simulink model "LAB3_SIMULINK_NO1_EBORA"  (R2023b)
settings: Solver=VariableStepAuto  StartTime=0.0  StopTime=20  RelTol=1e-3
values from neighbouring files (symbols this model uses):
  G1_den = [1 0 0]    [LAB3_MATLAB_NO1_BUENAFE.m]    (also in LAB3_MATLAB_NO2_RAGO.m)
  G1_num = [1]    [LAB3_MATLAB_NO1_BUENAFE.m]    (also in LAB3_MATLAB_NO2_RAGO.m)
  G2_den = [1 1]    [LAB3_MATLAB_NO1_BUENAFE.m]    (also in LAB3_MATLAB_NO2_RAGO.m)
  G2_num = [1]    [LAB3_MATLAB_NO1_BUENAFE.m]    (also in LAB3_MATLAB_NO2_RAGO.m)
  G3_den = [1 0]    [LAB3_MATLAB_NO1_BUENAFE.m]    (also in LAB3_MATLAB_NO2_RAGO.m)
  G3_num = [1]    [LAB3_MATLAB_NO1_BUENAFE.m]    (also in LAB3_MATLAB_NO2_RAGO.m)
  H1_den = [1 0]    [LAB3_MATLAB_NO1_BUENAFE.m]    (also in LAB3_MATLAB_NO2_RAGO.m)
  H1_num = [1]    [LAB3_MATLAB_NO1_BUENAFE.m]    (also in LAB3_MATLAB_NO2_RAGO.m)
  H2_den = [1 -1]    [LAB3_MATLAB_NO1_BUENAFE.m]    (also in LAB3_MATLAB_NO2_RAGO.m)
  H2_num = [1]    [LAB3_MATLAB_NO1_BUENAFE.m]    (also in LAB3_MATLAB_NO2_RAGO.m)
  H3_den = [1 -2]    [LAB3_MATLAB_NO1_BUENAFE.m]    (also in LAB3_MATLAB_NO2_RAGO.m)
  H3_num = [1]    [LAB3_MATLAB_NO1_BUENAFE.m]    (also in LAB3_MATLAB_NO2_RAGO.m)
  TF_den = conv(TF_num_down,TF_den_up)    [LAB3_MATLAB_NO1_BUENAFE.m]    (also in LAB3_MATLAB_NO2_RAGO.m)
  TF_num = conv(TF_num_up,TF_den_down)    [LAB3_MATLAB_NO1_BUENAFE.m]    (also in LAB3_MATLAB_NO2_RAGO.m)
settings Model: Creator=Troy  LastModifiedBy=Troy

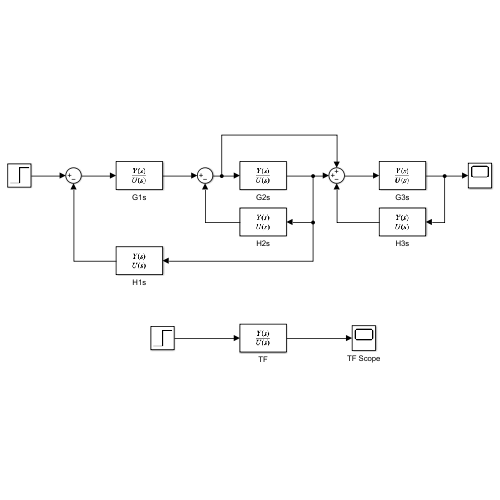
[thumbnail: Simulink's stored preview of the top-level diagram]
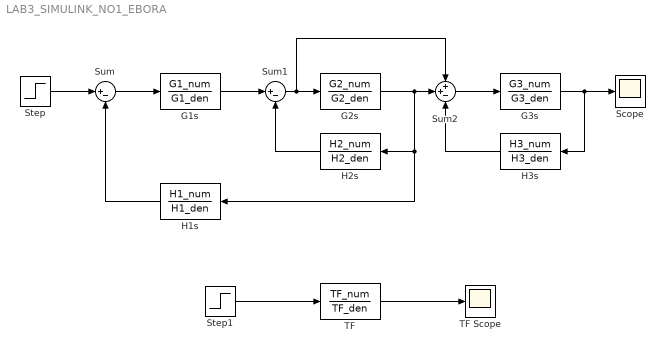
== system LAB3_SIMULINK_NO1_EBORA ==
  G1s : TransferFcn  Numerator=G1_num  Denominator=G1_den
  G2s : TransferFcn  Numerator=G2_num  Denominator=G2_den
  G3s : TransferFcn  Numerator=G3_num  Denominator=G3_den
  H1s : TransferFcn  Numerator=H1_num  Denominator=H1_den
  H2s : TransferFcn  Numerator=H2_num  Denominator=H2_den
  H3s : TransferFcn  Numerator=H3_num  Denominator=H3_den
  Scope : Scope
  Step : Step  Time=0  SampleTime=0
  Step1 : Step  Time=0  SampleTime=0
  Sum : Sum  Inputs=|+-
  Sum1 : Sum  Inputs=|+-
  Sum2 : Sum  Inputs=++-
  TF : TransferFcn  Numerator=TF_num  Denominator=TF_den
  TF Scope : Scope
  wires:
  Step/1 -> Sum/1
  Sum/1 -> G1s/1
  H1s/1 -> Sum/2
  G1s/1 -> Sum1/1
  Sum1/1 -> Sum2/1, G2s/1
  Sum2/1 -> G3s/1
  G2s/1 -> H1s/1, H2s/1, Sum2/2
  G3s/1 -> H3s/1, Scope/1
  H2s/1 -> Sum1/2
  H3s/1 -> Sum2/3
  Step1/1 -> TF/1
  TF/1 -> TF Scope/1
